simulink model "ModeAdjust"  (R2018b)
settings: Solver=FixedStepDiscrete  StartTime=0.0  StopTime=inf  FixedStep=0.01  RelTol=1e-3
undefined symbols (not defined in the file or in its folder): IfKeSMSbSeatMovBkRclnEnable_Val, IfKeSMSbSeatMovFrwdBkwdEnable_Val, IfKeSMSbSeatMovFtrstEnable_Val, IfKeSMSbSeatMovHdrstFrwdBkwdEnable_Val, IfKeSMSbSeatMovHdUpwdDnwdEnable_Val, IfKeSMSbSeatMovLgrstEnable_Val, IfKeSMSbSeatMovLtwdRtwdEnable_Val, IfVeSMSeStNumConfig, KeSMSbArmscreenMovEnable_Val, KeSMSbSeatMovLgrstExpdEnable_Val, KeSMSuFirstRwStBackPosDelta_Val, KeSMSuFirstRwStBackPosTolr_Val, KeSMSuFirstRwStCushFrntPosDelta_Val, KeSMSuFirstRwStCushFrntPosTolr_Val, KeSMSuFirstRwStCushRePosDelta_Val, KeSMSuFirstRwStCushRePosTolr_Val, KeSMSuFirstRwStFootrestPosDelta_Val, KeSMSuFirstRwStFootrestPosTolr_Val, KeSMSuFirstRwStFwdBkwdPosDelta_Val, KeSMSuFirstRwStFwdBkwdPosTolr_Val, KeSMSuMdMotFinshdTm_Val, KeSMSuMdRetryTm1_Val, KeSMSuModeReqDurgTm_Val, KeSMSuSecRwStArmTochPosDelta_Val, KeSMSuSecRwStArmTochPosTolr_Val, KeSMSuSecRwStBackPosDelta_Val, KeSMSuSecRwStBackPosTolr_Val, KeSMSuSecRwStFtrstUpwdDnwdPosDelta_Val, KeSMSuSecRwStFtrstUpwdDnwdPosTolr_Val, KeSMSuSecRwStFwdBkwdPosDelta_Val, KeSMSuSecRwStFwdBkwdPosTolr_Val, KeSMSuSecRwStHeadrestFwdBkwdPosDelta_Val, KeSMSuSecRwStHeadrestFwdBkwdPosTolr_Val, KeSMSuSecRwStHeadrestUpwdDwnwdPosDelta_Val, KeSMSuSecRwStHeadrestUpwdDwnwdPosTolr_Val, KeSMSuSecRwStLegrestInOutPosDelta_Val, KeSMSuSecRwStLegrestInOutPosTolr_Val, KeSMSuSecRwStLegrestUpwdDwnwdPosDelta_Val, KeSMSuSecRwStLegrestUpwdDwnwdPosTolr_Val, KeSMSuSecRwStLwdRwdPosDelta_Val, KeSMSuSecRwStLwdRwdPosTolr_Val, KeSMSuSecRwStVIPFtrstRefAngle_Val, KeSMSuThirdRwStFwdBkwdPosDelta_Val, KeSMSuThirdRwStFwdBkwdPosTolr_Val, KeSMSuThrdRwCushFoldPosDelta_Val, KeSMSuThrdRwCushFoldPosTolr_Val, KeSMSuThrdRwStBackPosDelta_Val, KeSMSuThrdRwStBackPosTolr_Val, KeSMSw4SLegrstCloseMdSecRwLtStFtrstUpwdDnwdPos_Val, KeSMSw4SLegrstCloseMdSecRwLtStFtrstUpwdDnwdPosMax_Val, KeSMSw4SLegrstCloseMdSecRwLtStFtrstUpwdDnwdPosMin_Val, KeSMSw4SLegrstCloseMdSecRwLtStLgrstOtwdInwdPos_Val, KeSMSw4SLegrstCloseMdSecRwLtStLgrstOtwdInwdPosMax_Val, KeSMSw4SLegrstCloseMdSecRwLtStLgrstOtwdInwdPosMin_Val, KeSMSw4SLegrstCloseMdSecRwLtStLgrstUpwdDnwdPos_Val, KeSMSw4SLegrstCloseMdSecRwLtStLgrstUpwdDnwdPosMax_Val, KeSMSw4SLegrstCloseMdSecRwLtStLgrstUpwdDnwdPosMin_Val, KeSMSw4SLegrstCloseMdSecRwRtStFtrstUpwdDnwdPos_Val, KeSMSw4SLegrstCloseMdSecRwRtStFtrstUpwdDnwdPosMax_Val, KeSMSw4SLegrstCloseMdSecRwRtStFtrstUpwdDnwdPosMin_Val ... (+1138)
libraries: Lib x401
(part 30 of 35)

== system ModeAdjust/ModeAdjustRunnable_sys/ModeAdjust/ArrivedAtTargetPosChk/Recovery4s/R2Lt ==
  SecRwLtStsPoss : Inport
  ModeStCalib_2L : Inport  Port=2
  StConfig : Inport  Port=3
  SecRwLtStsPoss4s : Inport  Port=4
  StConfig4s : Inport  Port=5
  SecRwLtStPossV : Inport  Port=6
  SecRwLtStPossV4s : Inport  Port=7
  Lt4sHightIndex : Inport  Port=8
  PosDeltaCalib : Inport  Port=9
  Bus Creator{,1..6} (7 alike) : BusCreator  Inputs=9
  Bus Selector : BusSelector  OutputSignals=IfVeSMSuSecRwLtStBkReclnUpwdDnwdPos_Val_read,IfVeSMSuSecRwLtStFrwdBkwdPos_Val_read,IfVeSMSuSecRwLtStHPassStUpwdDnwdPos_Val_read,IfVeSMSuSecRwLtStLgrstUpwdDnwdPos_Val_read,IfVeSMSuSecRwLtStLtwdRtwdPos_Val_read,IfVeSMSuSecRwLtStArmScrnPos_Val_read
  Bus Selector1 : BusSelector  OutputSignals=IfVeSMSuSecRwLtStLgrstOtwdInwdPos_Val_read,IfVeSMSuRrLtStFtUpwdDnwdPos_Val_read,IfVeSMSuSecRwLtStHdrstFrwdBkwdPos_Val_read
  Bus Selector2 : BusSelector  OutputSignals=BkReclnUpwdDnwdPosMax,BkReclnUpwdDnwdPosMin,LgrstUpwdPosMax,LgrstUpwdPosMin,FtrstUpwdDnwdPosMax,FtrstUpwdDnwdPosMin
  Bus Selector3 : BusSelector  OutputSignals=RecvyLSecRwLtSt
  Bus Selector4 : BusSelector  OutputSignals=BkReclnUpwdDnwdMovConfig,ArmTouchMovConfig,FrwdBkwdMovConfig,LgrstUpwdMovConfig,LtwdRtwdMovConfig
  Bus Selector5 : BusSelector  OutputSignals=LgrstExpdMovConfig,FtrstMovConfig,HdrstUpwdDnwdMovConfig,HdrstFrwdBkwdMovConfig
  Bus Selector6 : BusSelector  OutputSignals=IfVeSMSuSecRwLtStBkReclnUpwdDnwdPosV_Val_read,IfVeSMSuSecRwLtStFrwdBkwdPosV_Val_read,IfVeSMSuSecRwLtStHPassStUpwdDnwdPosV_Val_read,IfVeSMSuSecRwLtStLgrstUpwdDnwdPosV_Val_read,IfVeSMSuSecRwLtStLtwdRtwdPosV_Val_read,IfVeSMSuSecRwLtStArmScrnPosV_Val_read
  Bus Selector7 : BusSelector  OutputSignals=IfVeSMSuSecRwLtStLgrstOtwdInwdPosV_Val_read,IfVeSMSuRrLtStFtUpwdDnwdPosV_Val_read,IfVeSMSuSecRwLtStHdrstFrwdBkwdPosV_Val_read
  Bus Selector8 : BusSelector  OutputSignals=HdrstUpwdDnwdPosMax,HdrstUpwdDnwdPosMin,HdrstFrwdBkwdnwdPosMax,HdrstFrwdBkwdnwdPosMin,LgrstOtwdInwdPosMax,LgrstOtwdInwdPosMin
  Bus Selector9 : BusSelector  OutputSignals=KeSMSuSecRwStHeadrestFwdBkwdPosDelta_Val,KeSMSuSecRwStHeadrestUpwdDwnwdPosDelta_Val,KeSMSuSecRwStLegrestInOutPosDelta_Val,KeSMSuSecRwStFtrstUpwdDnwdPosDelta_Val,KeSMSuSecRwStBackPosDelta_Val,KeSMSuSecRwStLegrestUpwdDwnwdPosDelta_Val
  CheckAtPos{,1..5} (6 alike) : Lib/CheckAtPos  SystemSampleTime=-1
  Constant{1..12} (12 alike) : Constant  Value=0  OutDataTypeStr=boolean
  IsArrivedTarZone{,1..5} (6 alike) : Lib/CommonUsed/IniPosjudg/Subsystem2  SystemSampleTime=-1
  Logical Operator9 : Logic  Inputs=6  AllPortsSameDT=off  OutDataTypeStr=boolean
  Multiport Switch : MultiPortSwitch  DataPortOrder=Zero-based contiguous  Inputs=7  DiagnosticForDefault=None  zeroidx=on
  PA_KeSMSw4sRecoveryMDSecRwLtStHdrstFrwdBkwdPosMax_160_Val : Constant  Value=KeSMSw4sRecoveryMDSecRwLtStHdrstFrwdBkwdPosMax_160_Val
  PA_KeSMSw4sRecoveryMDSecRwLtStHdrstFrwdBkwdPosMax_165_Val : Constant  Value=KeSMSw4sRecoveryMDSecRwLtStHdrstFrwdBkwdPosMax_165_Val
  PA_KeSMSw4sRecoveryMDSecRwLtStHdrstFrwdBkwdPosMax_170_Val : Constant  Value=KeSMSw4sRecoveryMDSecRwLtStHdrstFrwdBkwdPosMax_170_Val
  PA_KeSMSw4sRecoveryMDSecRwLtStHdrstFrwdBkwdPosMax_175_Val : Constant  Value=KeSMSw4sRecoveryMDSecRwLtStHdrstFrwdBkwdPosMax_175_Val
  PA_KeSMSw4sRecoveryMDSecRwLtStHdrstFrwdBkwdPosMax_180_Val : Constant  Value=KeSMSw4sRecoveryMDSecRwLtStHdrstFrwdBkwdPosMax_180_Val
  PA_KeSMSw4sRecoveryMDSecRwLtStHdrstFrwdBkwdPosMax_Below160_Val : Constant  Value=KeSMSw4sRecoveryMDSecRwLtStHdrstFrwdBkwdPosMax_Below160_Val
  PA_KeSMSw4sRecoveryMDSecRwLtStHdrstFrwdBkwdPosMax_Over180_Val : Constant  Value=KeSMSw4sRecoveryMDSecRwLtStHdrstFrwdBkwdPosMax_Over180_Val
  PA_KeSMSw4sRecoveryMDSecRwLtStHdrstFrwdBkwdPosMin_160_Val : Constant  Value=KeSMSw4sRecoveryMDSecRwLtStHdrstFrwdBkwdPosMin_160_Val
  PA_KeSMSw4sRecoveryMDSecRwLtStHdrstFrwdBkwdPosMin_165_Val : Constant  Value=KeSMSw4sRecoveryMDSecRwLtStHdrstFrwdBkwdPosMin_165_Val
  PA_KeSMSw4sRecoveryMDSecRwLtStHdrstFrwdBkwdPosMin_170_Val : Constant  Value=KeSMSw4sRecoveryMDSecRwLtStHdrstFrwdBkwdPosMin_170_Val
  PA_KeSMSw4sRecoveryMDSecRwLtStHdrstFrwdBkwdPosMin_175_Val : Constant  Value=KeSMSw4sRecoveryMDSecRwLtStHdrstFrwdBkwdPosMin_175_Val
  PA_KeSMSw4sRecoveryMDSecRwLtStHdrstFrwdBkwdPosMin_180_Val : Constant  Value=KeSMSw4sRecoveryMDSecRwLtStHdrstFrwdBkwdPosMin_180_Val
  PA_KeSMSw4sRecoveryMDSecRwLtStHdrstFrwdBkwdPosMin_Below160_Val : Constant  Value=KeSMSw4sRecoveryMDSecRwLtStHdrstFrwdBkwdPosMin_Below160_Val
  PA_KeSMSw4sRecoveryMDSecRwLtStHdrstFrwdBkwdPosMin_Over180_Val : Constant  Value=KeSMSw4sRecoveryMDSecRwLtStHdrstFrwdBkwdPosMin_Over180_Val
  PA_KeSMSw4sRecoveryMDSecRwLtStHdrstFrwdBkwdPos_160_Val : Constant  Value=KeSMSw4sRecoveryMDSecRwLtStHdrstFrwdBkwdPos_160_Val
  PA_KeSMSw4sRecoveryMDSecRwLtStHdrstFrwdBkwdPos_165_Val : Constant  Value=KeSMSw4sRecoveryMDSecRwLtStHdrstFrwdBkwdPos_165_Val
  PA_KeSMSw4sRecoveryMDSecRwLtStHdrstFrwdBkwdPos_170_Val : Constant  Value=KeSMSw4sRecoveryMDSecRwLtStHdrstFrwdBkwdPos_170_Val
  PA_KeSMSw4sRecoveryMDSecRwLtStHdrstFrwdBkwdPos_175_Val : Constant  Value=KeSMSw4sRecoveryMDSecRwLtStHdrstFrwdBkwdPos_175_Val
  PA_KeSMSw4sRecoveryMDSecRwLtStHdrstFrwdBkwdPos_180_Val : Constant  Value=KeSMSw4sRecoveryMDSecRwLtStHdrstFrwdBkwdPos_180_Val
  PA_KeSMSw4sRecoveryMDSecRwLtStHdrstFrwdBkwdPos_Below160_Val : Constant  Value=KeSMSw4sRecoveryMDSecRwLtStHdrstFrwdBkwdPos_Below160_Val
  PA_KeSMSw4sRecoveryMDSecRwLtStHdrstFrwdBkwdPos_Over180_Val : Constant  Value=KeSMSw4sRecoveryMDSecRwLtStHdrstFrwdBkwdPos_Over180_Val
  PA_KeSMSw4sRecoveryMDSecRwLtStHdrstUpwdDnwdPosMax_160_Val : Constant  Value=KeSMSw4sRecoveryMDSecRwLtStHdrstUpwdDnwdPosMax_160_Val
  PA_KeSMSw4sRecoveryMDSecRwLtStHdrstUpwdDnwdPosMax_165_Val : Constant  Value=KeSMSw4sRecoveryMDSecRwLtStHdrstUpwdDnwdPosMax_165_Val
  PA_KeSMSw4sRecoveryMDSecRwLtStHdrstUpwdDnwdPosMax_170_Val : Constant  Value=KeSMSw4sRecoveryMDSecRwLtStHdrstUpwdDnwdPosMax_170_Val
  PA_KeSMSw4sRecoveryMDSecRwLtStHdrstUpwdDnwdPosMax_175_Val : Constant  Value=KeSMSw4sRecoveryMDSecRwLtStHdrstUpwdDnwdPosMax_175_Val
  PA_KeSMSw4sRecoveryMDSecRwLtStHdrstUpwdDnwdPosMax_180_Val : Constant  Value=KeSMSw4sRecoveryMDSecRwLtStHdrstUpwdDnwdPosMax_180_Val
  PA_KeSMSw4sRecoveryMDSecRwLtStHdrstUpwdDnwdPosMax_Below160_Val : Constant  Value=KeSMSw4sRecoveryMDSecRwLtStHdrstUpwdDnwdPosMax_Below160_Val
  PA_KeSMSw4sRecoveryMDSecRwLtStHdrstUpwdDnwdPosMax_Over180_Val : Constant  Value=KeSMSw4sRecoveryMDSecRwLtStHdrstUpwdDnwdPosMax_Over180_Val
  PA_KeSMSw4sRecoveryMDSecRwLtStHdrstUpwdDnwdPosMin_160_Val : Constant  Value=KeSMSw4sRecoveryMDSecRwLtStHdrstUpwdDnwdPosMin_160_Val
  PA_KeSMSw4sRecoveryMDSecRwLtStHdrstUpwdDnwdPosMin_165_Val : Constant  Value=KeSMSw4sRecoveryMDSecRwLtStHdrstUpwdDnwdPosMin_165_Val
  PA_KeSMSw4sRecoveryMDSecRwLtStHdrstUpwdDnwdPosMin_170_Val : Constant  Value=KeSMSw4sRecoveryMDSecRwLtStHdrstUpwdDnwdPosMin_170_Val
  PA_KeSMSw4sRecoveryMDSecRwLtStHdrstUpwdDnwdPosMin_175_Val : Constant  Value=KeSMSw4sRecoveryMDSecRwLtStHdrstUpwdDnwdPosMin_175_Val
  PA_KeSMSw4sRecoveryMDSecRwLtStHdrstUpwdDnwdPosMin_180_Val : Constant  Value=KeSMSw4sRecoveryMDSecRwLtStHdrstUpwdDnwdPosMin_180_Val
  PA_KeSMSw4sRecoveryMDSecRwLtStHdrstUpwdDnwdPosMin_Below160_Val : Constant  Value=KeSMSw4sRecoveryMDSecRwLtStHdrstUpwdDnwdPosMin_Below160_Val
  PA_KeSMSw4sRecoveryMDSecRwLtStHdrstUpwdDnwdPosMin_Over180_Val : Constant  Value=KeSMSw4sRecoveryMDSecRwLtStHdrstUpwdDnwdPosMin_Over180_Val
  PA_KeSMSw4sRecoveryMDSecRwLtStHdrstUpwdDnwdPos_160_Val : Constant  Value=KeSMSw4sRecoveryMDSecRwLtStHdrstUpwdDnwdPos_160_Val
  PA_KeSMSw4sRecoveryMDSecRwLtStHdrstUpwdDnwdPos_165_Val : Constant  Value=KeSMSw4sRecoveryMDSecRwLtStHdrstUpwdDnwdPos_165_Val
  PA_KeSMSw4sRecoveryMDSecRwLtStHdrstUpwdDnwdPos_170_Val : Constant  Value=KeSMSw4sRecoveryMDSecRwLtStHdrstUpwdDnwdPos_170_Val
  PA_KeSMSw4sRecoveryMDSecRwLtStHdrstUpwdDnwdPos_175_Val : Constant  Value=KeSMSw4sRecoveryMDSecRwLtStHdrstUpwdDnwdPos_175_Val
  PA_KeSMSw4sRecoveryMDSecRwLtStHdrstUpwdDnwdPos_180_Val : Constant  Value=KeSMSw4sRecoveryMDSecRwLtStHdrstUpwdDnwdPos_180_Val
  PA_KeSMSw4sRecoveryMDSecRwLtStHdrstUpwdDnwdPos_Below160_Val : Constant  Value=KeSMSw4sRecoveryMDSecRwLtStHdrstUpwdDnwdPos_Below160_Val
  PA_KeSMSw4sRecoveryMDSecRwLtStHdrstUpwdDnwdPos_Over180_Val : Constant  Value=KeSMSw4sRecoveryMDSecRwLtStHdrstUpwdDnwdPos_Over180_Val
  PA_KeSMSw4sRecoveryMDSecRwLtStLgrstOtwdInwdPosMax_160_Val : Constant  Value=KeSMSw4sRecoveryMDSecRwLtStLgrstOtwdInwdPosMax_160_Val
  PA_KeSMSw4sRecoveryMDSecRwLtStLgrstOtwdInwdPosMax_165_Val : Constant  Value=KeSMSw4sRecoveryMDSecRwLtStLgrstOtwdInwdPosMax_165_Val
  PA_KeSMSw4sRecoveryMDSecRwLtStLgrstOtwdInwdPosMax_170_Val : Constant  Value=KeSMSw4sRecoveryMDSecRwLtStLgrstOtwdInwdPosMax_170_Val
  PA_KeSMSw4sRecoveryMDSecRwLtStLgrstOtwdInwdPosMax_175_Val : Constant  Value=KeSMSw4sRecoveryMDSecRwLtStLgrstOtwdInwdPosMax_175_Val
  PA_KeSMSw4sRecoveryMDSecRwLtStLgrstOtwdInwdPosMax_180_Val : Constant  Value=KeSMSw4sRecoveryMDSecRwLtStLgrstOtwdInwdPosMax_180_Val
  PA_KeSMSw4sRecoveryMDSecRwLtStLgrstOtwdInwdPosMax_Below160_Val : Constant  Value=KeSMSw4sRecoveryMDSecRwLtStLgrstOtwdInwdPosMax_Below160_Val
  PA_KeSMSw4sRecoveryMDSecRwLtStLgrstOtwdInwdPosMax_Over180_Val : Constant  Value=KeSMSw4sRecoveryMDSecRwLtStLgrstOtwdInwdPosMax_Over180_Val
  PA_KeSMSw4sRecoveryMDSecRwLtStLgrstOtwdInwdPosMin_160_Val : Constant  Value=KeSMSw4sRecoveryMDSecRwLtStLgrstOtwdInwdPosMin_160_Val
  PA_KeSMSw4sRecoveryMDSecRwLtStLgrstOtwdInwdPosMin_165_Val : Constant  Value=KeSMSw4sRecoveryMDSecRwLtStLgrstOtwdInwdPosMin_165_Val
  PA_KeSMSw4sRecoveryMDSecRwLtStLgrstOtwdInwdPosMin_170_Val : Constant  Value=KeSMSw4sRecoveryMDSecRwLtStLgrstOtwdInwdPosMin_170_Val
  PA_KeSMSw4sRecoveryMDSecRwLtStLgrstOtwdInwdPosMin_175_Val : Constant  Value=KeSMSw4sRecoveryMDSecRwLtStLgrstOtwdInwdPosMin_175_Val
  PA_KeSMSw4sRecoveryMDSecRwLtStLgrstOtwdInwdPosMin_180_Val : Constant  Value=KeSMSw4sRecoveryMDSecRwLtStLgrstOtwdInwdPosMin_180_Val
  PA_KeSMSw4sRecoveryMDSecRwLtStLgrstOtwdInwdPosMin_Below160_Val : Constant  Value=KeSMSw4sRecoveryMDSecRwLtStLgrstOtwdInwdPosMin_Below160_Val
  PA_KeSMSw4sRecoveryMDSecRwLtStLgrstOtwdInwdPosMin_Over180_Val : Constant  Value=KeSMSw4sRecoveryMDSecRwLtStLgrstOtwdInwdPosMin_Over180_Val
  PA_KeSMSw4sRecoveryMDSecRwLtStLgrstOtwdInwdPos_160_Val : Constant  Value=KeSMSw4sRecoveryMDSecRwLtStLgrstOtwdInwdPos_160_Val
  PA_KeSMSw4sRecoveryMDSecRwLtStLgrstOtwdInwdPos_165_Val : Constant  Value=KeSMSw4sRecoveryMDSecRwLtStLgrstOtwdInwdPos_165_Val
  PA_KeSMSw4sRecoveryMDSecRwLtStLgrstOtwdInwdPos_170_Val : Constant  Value=KeSMSw4sRecoveryMDSecRwLtStLgrstOtwdInwdPos_170_Val
  PA_KeSMSw4sRecoveryMDSecRwLtStLgrstOtwdInwdPos_175_Val : Constant  Value=KeSMSw4sRecoveryMDSecRwLtStLgrstOtwdInwdPos_175_Val
  PA_KeSMSw4sRecoveryMDSecRwLtStLgrstOtwdInwdPos_180_Val : Constant  Value=KeSMSw4sRecoveryMDSecRwLtStLgrstOtwdInwdPos_180_Val
  PA_KeSMSw4sRecoveryMDSecRwLtStLgrstOtwdInwdPos_Below160_Val : Constant  Value=KeSMSw4sRecoveryMDSecRwLtStLgrstOtwdInwdPos_Below160_Val
  PA_KeSMSw4sRecoveryMDSecRwLtStLgrstOtwdInwdPos_Over180_Val : Constant  Value=KeSMSw4sRecoveryMDSecRwLtStLgrstOtwdInwdPos_Over180_Val
  R2Lt_ArrivedTarPos : Outport
  Calib_Recoery4sLAdpt : Outport  Port=2
  wires:
  Bus Selector5/2 -> [FtrstMovConfig]  "<FtrstMovConfig>"
  Bus Selector5/1 -> [LgrstExpdMovConfig]  "<LgrstExpdMovConfig>"
  Bus Selector5/3 -> [HdrstMovConfig]  "<HdrstUpwdDnwdMovConfig>"
  StConfig4s/1 -> Bus Selector5/1
  IsArrivedTarZone4/1 -> [Step1_5_ArrivedTarPos]
  [KeSMSuSecRwStLegrestInOutPosDelta_Val] -> IsArrivedTarZone4/3
  [SecRwLtStLgrstOtwdInwdPos] -> IsArrivedTarZone4/1
  [K_LgrstOtwdInwdPos_Max] -> IsArrivedTarZone4/4
  [K_LgrstOtwdInwdPos_Min] -> IsArrivedTarZone4/2
  IsArrivedTarZone3/1 -> [Step1_4_ArrivedTarPos]
  [K_FtrstUpwdDnwdPos_Max] -> IsArrivedTarZone3/4
  [K_FtrstUpwdDnwdPos_Min] -> IsArrivedTarZone3/2
  Bus Selector2/6 -> [K_FtrstUpwdDnwdPos_Min]  "<FtrstUpwdDnwdPosMin>"
  Bus Selector2/5 -> [K_FtrstUpwdDnwdPos_Max]  "<FtrstUpwdDnwdPosMax>"
  [IfVeSMSuRrLtStFtUpwdDnwdPos] -> IsArrivedTarZone3/1
  Bus Selector1/2 -> [IfVeSMSuRrLtStFtUpwdDnwdPos]  "<IfVeSMSuRrLtStFtUpwdDnwdPos_Val_read>"
  Bus Selector1/1 -> [SecRwLtStLgrstOtwdInwdPos]  "<IfVeSMSuSecRwLtStLgrstOtwdInwdPos_Val_read>"
  SecRwLtStsPoss4s/1 -> Bus Selector1/1
  [KeSMSuSecRwStFtrstUpwdDnwdPosDelta_Val] -> IsArrivedTarZone3/3
  [KeSMSuSecRwStHeadrestUpwdDwnwdPosDelta_Val] -> IsArrivedTarZone2/3
  [SecRwLtStHPassStUpwdDnwdPos] -> IsArrivedTarZone2/1
  [K_HdrstUpwdPosMin] -> IsArrivedTarZone2/2
  [K_HdrstUpwdPosMax] -> IsArrivedTarZone2/4
  Bus Selector4/1 -> [BkReclnUpwdDnwdMovConfig]  "<BkReclnUpwdDnwdMovConfig>"
  Bus Selector4/2 -> [ArmTouchMovConfig]  "<ArmTouchMovConfig>"
  Bus Selector4/4 -> [LgrstUpwdMovConfig]  "<LgrstUpwdMovConfig>"
  Bus Selector4/5 -> [LtwdRtwdMovConfig]  "<LtwdRtwdMovConfig>"
  Bus Selector4/3 -> [FrwdBkwdMovConfig]  "<FrwdBkwdMovConfig>"
  StConfig/1 -> Bus Selector4/1
  ModeStCalib_2L/1 -> Bus Selector3/1
  Bus Selector2/2 -> [K_BkReclnUpwdDnwdPosMin]  "<BkReclnUpwdDnwdPosMin>"
  Bus Selector3/1 -> Bus Selector2/1  "<RecvyLSecRwLtSt>"
  Bus Selector2/1 -> [K_BkReclnUpwdDnwdPosMax]  "<BkReclnUpwdDnwdPosMax>"
  Bus Selector2/3 -> [K_LgrstUpwdPosMax]  "<LgrstUpwdPosMax>"
  Bus Selector2/4 -> [K_LgrstUpwdPosMin]  "<LgrstUpwdPosMin>"
  [KeSMSuSecRwStLegrestUpwdDwnwdPosDelta_Val] -> IsArrivedTarZone1/3
  [K_LgrstUpwdPosMax] -> IsArrivedTarZone1/4
  [K_BkReclnUpwdDnwdPosMax] -> IsArrivedTarZone/4
  [KeSMSuSecRwStBackPosDelta_Val] -> IsArrivedTarZone/3
  Bus Selector/6 -> [SecRwLtStArmScrnPos]  "<IfVeSMSuSecRwLtStArmScrnPos_Val_read>"
  IsArrivedTarZone2/1 -> [Step1_3_ArrivedTarPos]
  Logical Operator9/1 -> R2Lt_ArrivedTarPos/1
  IsArrivedTarZone1/1 -> [Step1_2_ArrivedTarPos]
  [SecRwLtStLgrstUpwdDnwdPos] -> IsArrivedTarZone1/1
  [K_LgrstUpwdPosMin] -> IsArrivedTarZone1/2
  Bus Selector/1 -> [SecRwLtStBkReclnUpwdDnwdPos]  "<IfVeSMSuSecRwLtStBkReclnUpwdDnwdPos_Val_read>"
  Bus Selector/2 -> [SecRwLtStFrwdBkwdPos]  "<IfVeSMSuSecRwLtStFrwdBkwdPos_Val_read>"
  Bus Selector/4 -> [SecRwLtStLgrstUpwdDnwdPos]  "<IfVeSMSuSecRwLtStLgrstUpwdDnwdPos_Val_read>"
  Bus Selector/3 -> [SecRwLtStHPassStUpwdDnwdPos]  "<IfVeSMSuSecRwLtStHPassStUpwdDnwdPos_Val_read>"
  SecRwLtStsPoss/1 -> Bus Selector/1
  Bus Selector/5 -> [SecRwLtStLtwdRtwdPos]  "<IfVeSMSuSecRwLtStLtwdRtwdPos_Val_read>"
  [K_BkReclnUpwdDnwdPosMin] -> IsArrivedTarZone/2
  [SecRwLtStBkReclnUpwdDnwdPos] -> IsArrivedTarZone/1
  IsArrivedTarZone/1 -> [Step1_1_ArrivedTarPos]
  CheckAtPos2/1 -> Logical Operator9/3  "recv4sL_Step1_3_ArrivedTarPos"
  CheckAtPos1/1 -> Logical Operator9/2  "recv4sL_Step1_2_ArrivedTarPos"
  CheckAtPos3/1 -> Logical Operator9/4  "recv4sL_Step1_4_ArrivedTarPos"
  CheckAtPos/1 -> Logical Operator9/1  "recv4sL_Step1_1_ArrivedTarPos"
  CheckAtPos4/1 -> Logical Operator9/5  "recv4sL_Step1_5_ArrivedTarPos"
  [BkReclnUpwdDnwdMovConfig] -> CheckAtPos/1
  [Step1_1_ArrivedTarPos] -> CheckAtPos/3
  [LgrstUpwdMovConfig] -> CheckAtPos1/1
  [Step1_2_ArrivedTarPos] -> CheckAtPos1/3
  [HdrstMovConfig] -> CheckAtPos2/1
  [Step1_3_ArrivedTarPos] -> CheckAtPos2/3
  [FtrstMovConfig] -> CheckAtPos3/1
  [Step1_4_ArrivedTarPos] -> CheckAtPos3/3
  [LgrstExpdMovConfig] -> CheckAtPos4/1
  [Step1_5_ArrivedTarPos] -> CheckAtPos4/3
  Bus Selector7/2 -> [RrLtStFtUpwdDnwdPosV]  "<IfVeSMSuRrLtStFtUpwdDnwdPosV_Val_read>"
  SecRwLtStPossV4s/1 -> Bus Selector7/1
  Bus Selector7/1 -> [SecRwLtStLgrstOtwdInwdPosV]  "<IfVeSMSuSecRwLtStLgrstOtwdInwdPosV_Val_read>"
  Bus Selector6/1 -> [SecRwLtStBkReclnUpwdDnwdPosV]  "<IfVeSMSuSecRwLtStBkReclnUpwdDnwdPosV_Val_read>"
  SecRwLtStPossV/1 -> Bus Selector6/1
  Bus Selector6/4 -> [SecRwLtStLgrstUpwdDnwdPosV]  "<IfVeSMSuSecRwLtStLgrstUpwdDnwdPosV_Val_read>"
  Bus Selector6/5 -> [SecRwLtStLtwdRtwdPosV]  "<IfVeSMSuSecRwLtStLtwdRtwdPosV_Val_read>"
  Bus Selector6/6 -> [IfVeSMSuSecRwLtStArmScrnPosV]  "<IfVeSMSuSecRwLtStArmScrnPosV_Val_read>"
  Bus Selector6/3 -> [SecRwLtStHPassStUpwdDnwdPosV]  "<IfVeSMSuSecRwLtStHPassStUpwdDnwdPosV_Val_read>"
  Bus Selector6/2 -> [SecRwLtStFrwdBkwdPosV]  "<IfVeSMSuSecRwLtStFrwdBkwdPosV_Val_read>"
  [SecRwLtStBkReclnUpwdDnwdPosV] -> CheckAtPos/2
  [SecRwLtStHPassStUpwdDnwdPosV] -> CheckAtPos2/2
  [SecRwLtStLgrstUpwdDnwdPosV] -> CheckAtPos1/2
  [SecRwLtStLgrstOtwdInwdPosV] -> CheckAtPos4/2
  [RrLtStFtUpwdDnwdPosV] -> CheckAtPos3/2
  Constant1/1 -> CheckAtPos4/4
  Constant4/1 -> CheckAtPos4/5
  Constant2/1 -> CheckAtPos3/4
  Constant3/1 -> CheckAtPos3/5
  Constant5/1 -> CheckAtPos2/4
  Constant6/1 -> CheckAtPos2/5
  Constant7/1 -> CheckAtPos1/4
  Constant8/1 -> CheckAtPos1/5
  Constant9/1 -> CheckAtPos/4
  Constant10/1 -> CheckAtPos/5
  [SecRwLtStHdrstFrwdBkwdPos] -> IsArrivedTarZone5/1
  [K_HdrstFrwdBkwdnwdPosMin] -> IsArrivedTarZone5/2
  [HdrstFrwdBkwdMovConfig] -> CheckAtPos5/1
  Constant12/1 -> CheckAtPos5/4
  Constant11/1 -> CheckAtPos5/5
  [Step1_6_ArrivedTarPos] -> CheckAtPos5/3
  [KeSMSuSecRwStHeadrestFwdBkwdPosDelta_Val] -> IsArrivedTarZone5/3
  [K_HdrstFrwdBkwdnwdPosMax] -> IsArrivedTarZone5/4
  IsArrivedTarZone5/1 -> [Step1_6_ArrivedTarPos]
  [SecRwLtStHdrstFrwdBkwdPosV] -> CheckAtPos5/2
  CheckAtPos5/1 -> Logical Operator9/6  "recv4sL_Step1_6_ArrivedTarPos"
  Bus Selector5/4 -> [HdrstFrwdBkwdMovConfig]  "<HdrstFrwdBkwdMovConfig>"
  Bus Selector7/3 -> [SecRwLtStHdrstFrwdBkwdPosV]  "<IfVeSMSuSecRwLtStHdrstFrwdBkwdPosV_Val_read>"
  Bus Selector1/3 -> [SecRwLtStHdrstFrwdBkwdPos]  "<IfVeSMSuSecRwLtStHdrstFrwdBkwdPos_Val_read>"
  Lt4sHightIndex/1 -> Multiport Switch/1
  Multiport Switch/1 -> Bus Selector8/1, Calib_Recoery4sLAdpt/1
  Bus Creator/1 -> Multiport Switch/2  "Recovery4sLAdpt"
  Bus Selector8/1 -> [K_HdrstUpwdPosMax]  "<HdrstUpwdDnwdPosMax>"
  Bus Selector8/2 -> [K_HdrstUpwdPosMin]  "<HdrstUpwdDnwdPosMin>"
  Bus Selector8/4 -> [K_HdrstFrwdBkwdnwdPosMin]  "<HdrstFrwdBkwdnwdPosMin>"
  Bus Selector8/3 -> [K_HdrstFrwdBkwdnwdPosMax]  "<HdrstFrwdBkwdnwdPosMax>"
  PA_KeSMSw4sRecoveryMDSecRwLtStHdrstFrwdBkwdPosMin_Below160_Val/1 -> Bus Creator/9  "HdrstFrwdBkwdnwdPosMin"
  PA_KeSMSw4sRecoveryMDSecRwLtStLgrstOtwdInwdPosMin_Below160_Val/1 -> Bus Creator/6  "LgrstOtwdInwdPosMin"
  PA_KeSMSw4sRecoveryMDSecRwLtStLgrstOtwdInwdPosMax_Below160_Val/1 -> Bus Creator/5  "LgrstOtwdInwdPosMax"
  PA_KeSMSw4sRecoveryMDSecRwLtStHdrstFrwdBkwdPosMax_Below160_Val/1 -> Bus Creator/8  "HdrstFrwdBkwdnwdPosMax"
  PA_KeSMSw4sRecoveryMDSecRwLtStHdrstUpwdDnwdPosMin_Below160_Val/1 -> Bus Creator/3  "HdrstUpwdDnwdPosMin"
  PA_KeSMSw4sRecoveryMDSecRwLtStLgrstOtwdInwdPos_Below160_Val/1 -> Bus Creator/4  "LgrstOtwdInwdPos"
  PA_KeSMSw4sRecoveryMDSecRwLtStHdrstUpwdDnwdPosMax_Below160_Val/1 -> Bus Creator/2  "HdrstUpwdDnwdPosMax"
  PA_KeSMSw4sRecoveryMDSecRwLtStHdrstUpwdDnwdPos_Below160_Val/1 -> Bus Creator/1  "HdrstUpwdDnwdPos"
  PA_KeSMSw4sRecoveryMDSecRwLtStHdrstFrwdBkwdPos_Below160_Val/1 -> Bus Creator/7  "HdrstFrwdBkwdnwdPos"
  PA_KeSMSw4sRecoveryMDSecRwLtStLgrstOtwdInwdPos_160_Val/1 -> Bus Creator1/4  "LgrstOtwdInwdPos"
  PA_KeSMSw4sRecoveryMDSecRwLtStLgrstOtwdInwdPosMax_160_Val/1 -> Bus Creator1/5  "LgrstOtwdInwdPosMax"
  Bus Creator1/1 -> Multiport Switch/3  "Recovery4sLAdpt"
  PA_KeSMSw4sRecoveryMDSecRwLtStHdrstFrwdBkwdPosMin_160_Val/1 -> Bus Creator1/9  "HdrstFrwdBkwdnwdPosMin"
  PA_KeSMSw4sRecoveryMDSecRwLtStHdrstFrwdBkwdPosMax_160_Val/1 -> Bus Creator1/8  "HdrstFrwdBkwdnwdPosMax"
  PA_KeSMSw4sRecoveryMDSecRwLtStLgrstOtwdInwdPosMin_160_Val/1 -> Bus Creator1/6  "LgrstOtwdInwdPosMin"
  PA_KeSMSw4sRecoveryMDSecRwLtStHdrstUpwdDnwdPosMax_160_Val/1 -> Bus Creator1/2  "HdrstUpwdDnwdPosMax"
  PA_KeSMSw4sRecoveryMDSecRwLtStHdrstUpwdDnwdPosMin_160_Val/1 -> Bus Creator1/3  "HdrstUpwdDnwdPosMin"
  PA_KeSMSw4sRecoveryMDSecRwLtStHdrstUpwdDnwdPos_160_Val/1 -> Bus Creator1/1  "HdrstUpwdDnwdPos"
  PA_KeSMSw4sRecoveryMDSecRwLtStHdrstFrwdBkwdPos_160_Val/1 -> Bus Creator1/7  "HdrstFrwdBkwdnwdPos"
  PA_KeSMSw4sRecoveryMDSecRwLtStLgrstOtwdInwdPosMax_165_Val/1 -> Bus Creator2/5  "LgrstOtwdInwdPosMax"
  PA_KeSMSw4sRecoveryMDSecRwLtStLgrstOtwdInwdPos_165_Val/1 -> Bus Creator2/4  "LgrstOtwdInwdPos"
  Bus Creator2/1 -> Multiport Switch/4  "Recovery4sLAdpt"
  PA_KeSMSw4sRecoveryMDSecRwLtStHdrstUpwdDnwdPosMin_165_Val/1 -> Bus Creator2/3  "HdrstUpwdDnwdPosMin"
  PA_KeSMSw4sRecoveryMDSecRwLtStHdrstFrwdBkwdPos_165_Val/1 -> Bus Creator2/7  "HdrstFrwdBkwdnwdPos"
  PA_KeSMSw4sRecoveryMDSecRwLtStHdrstUpwdDnwdPosMax_165_Val/1 -> Bus Creator2/2  "HdrstUpwdDnwdPosMax"
  PA_KeSMSw4sRecoveryMDSecRwLtStHdrstFrwdBkwdPosMax_165_Val/1 -> Bus Creator2/8  "HdrstFrwdBkwdnwdPosMax"
  PA_KeSMSw4sRecoveryMDSecRwLtStHdrstFrwdBkwdPosMin_165_Val/1 -> Bus Creator2/9  "HdrstFrwdBkwdnwdPosMin"
  PA_KeSMSw4sRecoveryMDSecRwLtStLgrstOtwdInwdPosMin_165_Val/1 -> Bus Creator2/6  "LgrstOtwdInwdPosMin"
  PA_KeSMSw4sRecoveryMDSecRwLtStHdrstUpwdDnwdPos_165_Val/1 -> Bus Creator2/1  "HdrstUpwdDnwdPos"
  PA_KeSMSw4sRecoveryMDSecRwLtStHdrstFrwdBkwdPosMin_170_Val/1 -> Bus Creator3/9  "HdrstFrwdBkwdnwdPosMin"
  PA_KeSMSw4sRecoveryMDSecRwLtStHdrstFrwdBkwdPosMax_170_Val/1 -> Bus Creator3/8  "HdrstFrwdBkwdnwdPosMax"
  PA_KeSMSw4sRecoveryMDSecRwLtStHdrstFrwdBkwdPos_170_Val/1 -> Bus Creator3/7  "HdrstFrwdBkwdnwdPos"
  PA_KeSMSw4sRecoveryMDSecRwLtStHdrstUpwdDnwdPosMin_170_Val/1 -> Bus Creator3/3  "HdrstUpwdDnwdPosMin"
  PA_KeSMSw4sRecoveryMDSecRwLtStHdrstUpwdDnwdPosMax_170_Val/1 -> Bus Creator3/2  "HdrstUpwdDnwdPosMax"
  Bus Creator3/1 -> Multiport Switch/5  "Recovery4sLAdpt"
  PA_KeSMSw4sRecoveryMDSecRwLtStHdrstUpwdDnwdPos_170_Val/1 -> Bus Creator3/1  "HdrstUpwdDnwdPos"
  PA_KeSMSw4sRecoveryMDSecRwLtStLgrstOtwdInwdPos_170_Val/1 -> Bus Creator3/4  "LgrstOtwdInwdPos"
  PA_KeSMSw4sRecoveryMDSecRwLtStLgrstOtwdInwdPosMin_170_Val/1 -> Bus Creator3/6  "LgrstOtwdInwdPosMin"
  PA_KeSMSw4sRecoveryMDSecRwLtStLgrstOtwdInwdPosMax_170_Val/1 -> Bus Creator3/5  "LgrstOtwdInwdPosMax"
  Bus Creator4/1 -> Multiport Switch/6  "Recovery4sLAdpt"
  PA_KeSMSw4sRecoveryMDSecRwLtStLgrstOtwdInwdPos_175_Val/1 -> Bus Creator4/4  "LgrstOtwdInwdPos"
  PA_KeSMSw4sRecoveryMDSecRwLtStLgrstOtwdInwdPosMin_175_Val/1 -> Bus Creator4/6  "LgrstOtwdInwdPosMin"
  PA_KeSMSw4sRecoveryMDSecRwLtStHdrstUpwdDnwdPosMax_175_Val/1 -> Bus Creator4/2  "HdrstUpwdDnwdPosMax"
  PA_KeSMSw4sRecoveryMDSecRwLtStLgrstOtwdInwdPosMax_175_Val/1 -> Bus Creator4/5  "LgrstOtwdInwdPosMax"
  PA_KeSMSw4sRecoveryMDSecRwLtStHdrstUpwdDnwdPosMin_175_Val/1 -> Bus Creator4/3  "HdrstUpwdDnwdPosMin"
  PA_KeSMSw4sRecoveryMDSecRwLtStHdrstFrwdBkwdPosMax_175_Val/1 -> Bus Creator4/8  "HdrstFrwdBkwdnwdPosMax"
  PA_KeSMSw4sRecoveryMDSecRwLtStHdrstUpwdDnwdPos_175_Val/1 -> Bus Creator4/1  "HdrstUpwdDnwdPos"
  PA_KeSMSw4sRecoveryMDSecRwLtStHdrstFrwdBkwdPos_175_Val/1 -> Bus Creator4/7  "HdrstFrwdBkwdnwdPos"
  PA_KeSMSw4sRecoveryMDSecRwLtStHdrstFrwdBkwdPosMin_175_Val/1 -> Bus Creator4/9  "HdrstFrwdBkwdnwdPosMin"
  PA_KeSMSw4sRecoveryMDSecRwLtStLgrstOtwdInwdPos_180_Val/1 -> Bus Creator5/4  "LgrstOtwdInwdPos"
  PA_KeSMSw4sRecoveryMDSecRwLtStLgrstOtwdInwdPosMax_180_Val/1 -> Bus Creator5/5  "LgrstOtwdInwdPosMax"
  PA_KeSMSw4sRecoveryMDSecRwLtStHdrstUpwdDnwdPosMax_180_Val/1 -> Bus Creator5/2  "HdrstUpwdDnwdPosMax"
  Bus Creator5/1 -> Multiport Switch/7  "Recovery4sLAdpt"
  PA_KeSMSw4sRecoveryMDSecRwLtStHdrstFrwdBkwdPosMax_180_Val/1 -> Bus Creator5/8  "HdrstFrwdBkwdnwdPosMax"
  PA_KeSMSw4sRecoveryMDSecRwLtStHdrstFrwdBkwdPos_180_Val/1 -> Bus Creator5/7  "HdrstFrwdBkwdnwdPos"
  PA_KeSMSw4sRecoveryMDSecRwLtStLgrstOtwdInwdPosMin_180_Val/1 -> Bus Creator5/6  "LgrstOtwdInwdPosMin"
  PA_KeSMSw4sRecoveryMDSecRwLtStHdrstFrwdBkwdPosMin_180_Val/1 -> Bus Creator5/9  "HdrstFrwdBkwdnwdPosMin"
  PA_KeSMSw4sRecoveryMDSecRwLtStHdrstUpwdDnwdPos_180_Val/1 -> Bus Creator5/1  "HdrstUpwdDnwdPos"
  PA_KeSMSw4sRecoveryMDSecRwLtStHdrstUpwdDnwdPosMin_180_Val/1 -> Bus Creator5/3  "HdrstUpwdDnwdPosMin"
  PA_KeSMSw4sRecoveryMDSecRwLtStHdrstUpwdDnwdPosMax_Over180_Val/1 -> Bus Creator6/2  "HdrstUpwdDnwdPosMax"
  PA_KeSMSw4sRecoveryMDSecRwLtStHdrstUpwdDnwdPosMin_Over180_Val/1 -> Bus Creator6/3  "HdrstUpwdDnwdPosMin"
  PA_KeSMSw4sRecoveryMDSecRwLtStHdrstUpwdDnwdPos_Over180_Val/1 -> Bus Creator6/1  "HdrstUpwdDnwdPos"
  PA_KeSMSw4sRecoveryMDSecRwLtStLgrstOtwdInwdPosMin_Over180_Val/1 -> Bus Creator6/6  "LgrstOtwdInwdPosMin"
  PA_KeSMSw4sRecoveryMDSecRwLtStLgrstOtwdInwdPosMax_Over180_Val/1 -> Bus Creator6/5  "LgrstOtwdInwdPosMax"
  PA_KeSMSw4sRecoveryMDSecRwLtStLgrstOtwdInwdPos_Over180_Val/1 -> Bus Creator6/4  "LgrstOtwdInwdPos"
  PA_KeSMSw4sRecoveryMDSecRwLtStHdrstFrwdBkwdPosMin_Over180_Val/1 -> Bus Creator6/9  "HdrstFrwdBkwdnwdPosMin"
  PA_KeSMSw4sRecoveryMDSecRwLtStHdrstFrwdBkwdPosMax_Over180_Val/1 -> Bus Creator6/8  "HdrstFrwdBkwdnwdPosMax"
  PA_KeSMSw4sRecoveryMDSecRwLtStHdrstFrwdBkwdPos_Over180_Val/1 -> Bus Creator6/7  "HdrstFrwdBkwdnwdPos"
  Bus Creator6/1 -> Multiport Switch/8  "Recovery4sLAdpt"
  Bus Selector8/6 -> [K_LgrstOtwdInwdPos_Min]  "<LgrstOtwdInwdPosMin>"
  Bus Selector8/5 -> [K_LgrstOtwdInwdPos_Max]  "<LgrstOtwdInwdPosMax>"
  Bus Selector9/5 -> [KeSMSuSecRwStBackPosDelta_Val]  "<KeSMSuSecRwStBackPosDelta_Val>"
  Bus Selector9/4 -> [KeSMSuSecRwStFtrstUpwdDnwdPosDelta_Val]  "<KeSMSuSecRwStFtrstUpwdDnwdPosDelta_Val>"
  Bus Selector9/6 -> [KeSMSuSecRwStLegrestUpwdDwnwdPosDelta_Val]  "<KeSMSuSecRwStLegrestUpwdDwnwdPosDelta_Val>"
  Bus Selector9/2 -> [KeSMSuSecRwStHeadrestUpwdDwnwdPosDelta_Val]  "<KeSMSuSecRwStHeadrestUpwdDwnwdPosDelta_Val>"
  Bus Selector9/3 -> [KeSMSuSecRwStLegrestInOutPosDelta_Val]  "<KeSMSuSecRwStLegrestInOutPosDelta_Val>"
  Bus Selector9/1 -> [KeSMSuSecRwStHeadrestFwdBkwdPosDelta_Val]  "<KeSMSuSecRwStHeadrestFwdBkwdPosDelta_Val>"
  PosDeltaCalib/1 -> Bus Selector9/1
